simulink model "modificar_acc_compilar"  (R2013b)
settings: Solver=ode45  StartTime=0.0  StopTime=17000  RelTol=1e-3
undefined symbols (not defined in the file): internal_oor, misc_lib, pfb_coeff_gen_calc, xlfda_numerator, xlipgetpartsetting
libraries: xbsIndex_r4 x1539, xps_library x14, dspsigops x8, casper_library_misc x8, casper_library_delays x3, simulink x1
(part 4 of 15)

== system modificar_acc_compilar/acc_cntrl0 ==
  acc_len : Inport
  sync : Inport  Port=2
  rst : Inport  Port=3
  Logical : xbsIndex_r4/Logical  logical_function=OR  inputs=2  en=off  latency=0  precision=Full  arith_type=Unsigned  n_bits=8  bin_pt=2  align_bp=on  dbl_ovrd=off  block_type=logical
      settings: xl_area=[0, 0, 0, 0, 0, 0, 0]
  Register : xbsIndex_r4/Register  init=0  rst=on  en=on  dbl_ovrd=off  block_type=register
      settings: xl_area=[0, 0, 0, 0, 0, 0, 0]
  Relational5 : xbsIndex_r4/Relational  mode=a=b  en=off  latency=0  dbl_ovrd=off  block_type=relational
      settings: xl_area=[0, 0, 0, 0, 0, 0, 0]  block_version=10.1.3
  Shift : xbsIndex_r4/Shift  shift_dir=Left  shift_bits=chan_bits  en=off  latency=0  precision=Full  arith_type="Signed  (2's comp)"  n_bits=8  bin_pt=2  quantization=Truncate  overflow=Wrap  dbl_ovrd=off  block_type=shift
      settings: xl_area=[0, 0, 0, 0, 0, 0, 0]  block_version=10.1.3
  cntr : xbsIndex_r4/Counter  cnt_type=Free Running  cnt_to=Inf  operation=Up  start_count=1  cnt_by_val=1  arith_type=Unsigned  n_bits=32  bin_pt=0  load_pin=off  rst=on  en=off  explicit_period=on  period=1  dbl_ovrd=off  use_behavioral_HDL=on  implementation=Fabric  use_rpm=on  block_type=counter
      settings: xl_area=[0, 0, 0, 0, 0, 0, 0]
  edge_detect : Subsystem  AncestorBlock=casper_library_misc/edge_detect  mask(edge_detect){edge=Rising, polarity=Active High, x_in=[0 0.08 0.08 0.16 0.16 0.24 0.24 0.32 0.32 0.4], y_in=[-1 -1  1  1  1  1  1  1  1  1], x_out=[0.6 0.68 0.68 0.76 0.76 0.84 0.84 0.92 0.92 1], y_out=[-1 -1  1  1 -1 -1 -1 -1 -1 -1]}
      mask prompts: edge "Edge Type"; polarity "Output Polarity"; x_in "Input X Positions"; y_in "Input Y Positions"; x_out "Output X Positions"; y_out "Output Y Positions"
      mask help: Output is active for one-cycle after each edge of the specified type (i.e. rising, falling or both).
      mask init: same as modificar_acc_compilar/edge_detect1
      settings: AttributesFormatString=|
      | rising edges
      | active high
      mask Help: Output is active for one-cycle after each edge of the specified type (i.e. rising, falling, or both).  Latency is zero.
      mask TypeOptions edge: Rising | Falling | Both
      mask TypeOptions polarity: Active High | Active Low
      mask Display:
      | plot(x_in_num,0.5+y_in_num*0.2);
      | plot(x_out_num,0.5+y_out_num*0.2);
  pipeline15 : Subsystem  AncestorBlock=casper_library_delays/pipeline  mask(pipeline){latency=1}
      mask help:
      | An explicitly laid-out delay line to avoid mapping to SRL16s
      | for use in pipelining to help achieve timing closure.
      mask init:
      | pipeline_init(gcb,'latency',latency);
      settings: AttributesFormatString=Latency = %<latency>
      mask Display:
      | port_label('input', 1, 'd');
      | port_label('output', 1, 'q');
      | disp(['Z^-', num2str(latency)]);
  new_acc : Outport
  wires:
  Shift/1 -> pipeline15/1(d)
  rst/1 -> Register/2
  sync/1 -> Register/3, Register/1
  Relational5/1 -> new_acc/1, Logical/2
  acc_len/1 -> Shift/1
  Logical/1 -> cntr/1
  Register/1 -> edge_detect/1(in)
  edge_detect/1(out) -> Logical/1
  pipeline15/1(q) -> Relational5/2
  cntr/1 -> Relational5/1

== system modificar_acc_compilar/acc_len ==
  io_delay : xbsIndex_r4/Delay  rst=off  infoeditControl=Selection of Reset will increase slice count due to use of real FFs and instead of SRLs  en=off  latency=0  dbl_ovrd=off  reg_retiming=on  block_type=delay
  modificar_acc_compilar_acc_len_user_data_out : xbsIndex_r4/Gateway In  gui_display_data_type=Fixed-point  arith_type=Unsigned  n_bits=32  bin_pt=0  preci_type=Single  exp_width=8  frac_width=24  quantization="Round  (unbiased: +/- Inf)"  overflow=Saturate  period=1  dbl_ovrd=off  timing_constraint=None  locs_specified=off  LOCs={}  UseAsADC=off  ADCChannel='1'  inherit_from_input=off  hdl_port=on  block_type=gatewayin
  reint1 : xbsIndex_r4/Reinterpret  force_arith_type=on  arith_type=Unsigned  force_bin_pt=on  bin_pt=0  block_type=reinterpret
  sim_1 : Constant  Value=0
  slice_reg : xbsIndex_r4/Slice  nbits=32  boolean_output=off  mode=Lower Bit Location + Width  bit1=0  base1=MSB of Input  bit0=0  base0=LSB of Input  dbl_ovrd=off  block_type=slice
  in_reg : Outport
  wires:
  modificar_acc_compilar_acc_len_user_data_out/1 -> io_delay/1
  sim_1/1 -> modificar_acc_compilar_acc_len_user_data_out/1
  io_delay/1 -> slice_reg/1
  slice_reg/1 -> reint1/1
  reint1/1 -> in_reg/1

== system modificar_acc_compilar/adc083000x2 ==
  adc0_sync_sim : Inport
  adc0_data_valid_sim : Inport  Port=2
  sim_adc0_data_in : Inport  Port=3
  adc0_sim : Subsystem  AncestorBlock=xps_library/ADCs/adc_sim  mask(adc_sim){nStreams=8, bit_width=8}
      mask prompts: nStreams "Number of Output Streams"; bit_width "Sample Bit Width"
      mask help:
      | This block simulates the behavior of a demuxed ADC, which takes
      | as input a waveform and returns digital samples in parallel at
      | a slower rate.
      |
      | This block is used to simulate the behavior
      mask init:
      | adc_sim_init(gcb, ...
      |     'nStreams', nStreams, ...
      |     'bit_width', bit_width);
  modificar_acc_compilar_adc083000x2_adc0_user_data_valid : xbsIndex_r4/Gateway In  gui_display_data_type=Fixed-point  arith_type=Unsigned  n_bits=1  bin_pt=0  preci_type=Single  exp_width=8  frac_width=24  quantization="Round  (unbiased: +/- Inf)"  overflow=Saturate  period=1  dbl_ovrd=off  timing_constraint=None  locs_specified=off  LOCs={}  UseAsADC=off  ADCChannel='1'  inherit_from_input=off  hdl_port=on  block_type=gatewayin
  modificar_acc_compilar_adc083000x2_adc0_user_outofrange : xbsIndex_r4/Gateway In  gui_display_data_type=Fixed-point  arith_type=Unsigned  n_bits=4  bin_pt=0  preci_type=Single  exp_width=8  frac_width=24  quantization="Round  (unbiased: +/- Inf)"  overflow=Saturate  period=1  dbl_ovrd=off  timing_constraint=None  locs_specified=off  LOCs={}  UseAsADC=off  ADCChannel='1'  inherit_from_input=off  hdl_port=on  block_type=gatewayin
  modificar_acc_compilar_adc083000x2_adc0_user_s{0..7} (8 alike) : xbsIndex_r4/Gateway In  gui_display_data_type=Fixed-point  arith_type=Unsigned  n_bits=8  bin_pt=0  preci_type=Single  exp_width=8  frac_width=24  quantization="Round  (unbiased: +/- Inf)"  overflow=Saturate  period=1  dbl_ovrd=off  timing_constraint=None  locs_specified=off  LOCs={}  UseAsADC=off  ADCChannel='1'  inherit_from_input=off  hdl_port=on  block_type=gatewayin
  modificar_acc_compilar_adc083000x2_adc0_user_s0_conv : xps_library/ADCs/conv  bit_width=8
  modificar_acc_compilar_adc083000x2_adc0_user_s1_conv : xps_library/ADCs/conv  bit_width=8
  modificar_acc_compilar_adc083000x2_adc0_user_s2_conv : xps_library/ADCs/conv  bit_width=8
  modificar_acc_compilar_adc083000x2_adc0_user_s3_conv : xps_library/ADCs/conv  bit_width=8
  modificar_acc_compilar_adc083000x2_adc0_user_s4_conv : xps_library/ADCs/conv  bit_width=8
  modificar_acc_compilar_adc083000x2_adc0_user_s5_conv : xps_library/ADCs/conv  bit_width=8
  modificar_acc_compilar_adc083000x2_adc0_user_s6_conv : xps_library/ADCs/conv  bit_width=8
  modificar_acc_compilar_adc083000x2_adc0_user_s7_conv : xps_library/ADCs/conv  bit_width=8
  modificar_acc_compilar_adc083000x2_adc0_user_sync : xbsIndex_r4/Gateway In  gui_display_data_type=Fixed-point  arith_type=Unsigned  n_bits=4  bin_pt=0  preci_type=Single  exp_width=8  frac_width=24  quantization="Round  (unbiased: +/- Inf)"  overflow=Saturate  period=1  dbl_ovrd=off  timing_constraint=None  locs_specified=off  LOCs={}  UseAsADC=off  ADCChannel='1'  inherit_from_input=off  hdl_port=on  block_type=gatewayin
  adc0_s0 : Outport
  adc0_s1 : Outport  Port=2
  adc0_s2 : Outport  Port=3
  adc0_s3 : Outport  Port=4
  adc0_s4 : Outport  Port=5
  adc0_s5 : Outport  Port=6
  adc0_s6 : Outport  Port=7
  adc0_s7 : Outport  Port=8
  adc0_sync : Outport  Port=9
  adc0_outofrange : Outport  Port=10
  adc0_data_valid : Outport  Port=11
  wires:
  sim_adc0_data_in/1 -> adc0_sim/1(sim_adc_data_in)
  adc0_sim/1(s0) -> modificar_acc_compilar_adc083000x2_adc0_user_s0/1
  modificar_acc_compilar_adc083000x2_adc0_user_s0/1 -> modificar_acc_compilar_adc083000x2_adc0_user_s0_conv/1
  modificar_acc_compilar_adc083000x2_adc0_user_s0_conv/1 -> adc0_s0/1
  adc0_sim/2(s1) -> modificar_acc_compilar_adc083000x2_adc0_user_s1/1
  modificar_acc_compilar_adc083000x2_adc0_user_s1/1 -> modificar_acc_compilar_adc083000x2_adc0_user_s1_conv/1
  modificar_acc_compilar_adc083000x2_adc0_user_s1_conv/1 -> adc0_s1/1
  adc0_sim/3(s2) -> modificar_acc_compilar_adc083000x2_adc0_user_s2/1
  modificar_acc_compilar_adc083000x2_adc0_user_s2/1 -> modificar_acc_compilar_adc083000x2_adc0_user_s2_conv/1
  modificar_acc_compilar_adc083000x2_adc0_user_s2_conv/1 -> adc0_s2/1
  adc0_sim/4(s3) -> modificar_acc_compilar_adc083000x2_adc0_user_s3/1
  modificar_acc_compilar_adc083000x2_adc0_user_s3/1 -> modificar_acc_compilar_adc083000x2_adc0_user_s3_conv/1
  modificar_acc_compilar_adc083000x2_adc0_user_s3_conv/1 -> adc0_s3/1
  adc0_sim/5(s4) -> modificar_acc_compilar_adc083000x2_adc0_user_s4/1
  modificar_acc_compilar_adc083000x2_adc0_user_s4/1 -> modificar_acc_compilar_adc083000x2_adc0_user_s4_conv/1
  modificar_acc_compilar_adc083000x2_adc0_user_s4_conv/1 -> adc0_s4/1
  adc0_sim/6(s5) -> modificar_acc_compilar_adc083000x2_adc0_user_s5/1
  modificar_acc_compilar_adc083000x2_adc0_user_s5/1 -> modificar_acc_compilar_adc083000x2_adc0_user_s5_conv/1
  modificar_acc_compilar_adc083000x2_adc0_user_s5_conv/1 -> adc0_s5/1
  adc0_sim/7(s6) -> modificar_acc_compilar_adc083000x2_adc0_user_s6/1
  modificar_acc_compilar_adc083000x2_adc0_user_s6/1 -> modificar_acc_compilar_adc083000x2_adc0_user_s6_conv/1
  modificar_acc_compilar_adc083000x2_adc0_user_s6_conv/1 -> adc0_s6/1
  adc0_sim/8(s7) -> modificar_acc_compilar_adc083000x2_adc0_user_s7/1
  modificar_acc_compilar_adc083000x2_adc0_user_s7/1 -> modificar_acc_compilar_adc083000x2_adc0_user_s7_conv/1
  modificar_acc_compilar_adc083000x2_adc0_user_s7_conv/1 -> adc0_s7/1
  adc0_sync_sim/1 -> modificar_acc_compilar_adc083000x2_adc0_user_sync/1
  modificar_acc_compilar_adc083000x2_adc0_user_sync/1 -> adc0_sync/1
  adc0_sim/9(of) -> modificar_acc_compilar_adc083000x2_adc0_user_outofrange/1
  modificar_acc_compilar_adc083000x2_adc0_user_outofrange/1 -> adc0_outofrange/1
  adc0_data_valid_sim/1 -> modificar_acc_compilar_adc083000x2_adc0_user_data_valid/1
  modificar_acc_compilar_adc083000x2_adc0_user_data_valid/1 -> adc0_data_valid/1

== system modificar_acc_compilar/adcsnap0 ==
  note: Generate stop
      | when in circular
      | capture mode
  note: Delay start
      | of capture
  note: ctrl:
      | bit0: Put a posedge here
      |         to enable a new capture.
      | bit1: ignore external trigger
      |         and trigger immediately.
      | bit2: ignore external write
      |         enable and capture on
      |         every FPGA clock.
      | bit3: continuously capture
      |         data until we get an
      |         external stop command.
  note: Offset in vector
      | from first element
      | captured, used
      | during circular capture
  note: Number of
      | bytes in
      | buffer and
      | done bit
  note: Number of valid
      | data samples to
      | skip after trigger
      | before starting
      | capture
  note: Value on vin
      | aligned with
      | first sample on
      | din captured
  din : Inport
  we : Inport  Port=2
  trig : Inport  Port=3
  add_del : xbsIndex_r4/Delay  rst=off  infoeditControl=Selection of Reset will increase slice count due to use of real FFs and instead of SRLs  en=off  latency=1  dbl_ovrd=off  reg_retiming=on  block_type=delay
      settings: block_version=11.4
  add_gen : Subsystem  AncestorBlock=casper_library_scopes/snapshot/add_gen  mask{counter_size=10+3+1, increment=8, nsamples=10, burst_size=0, use_dsp48=on}
      mask prompts: counter_size "Address counter size (2^?)"; increment "Address counter increment"; nsamples "Number of samples (2^?)"; burst_size "Burst size (2^?)"; use_dsp48 "dsp48 counter/s"
      mask init:
      | set_param(gcb,'LinkStatus','inactive');
      | if strcmp(use_dsp48,'on'),
      |     set_param([gcb,'/add_gen'],'implementation','DSP48');
      | else
      |     set_param([gcb,'/add_gen'],'implementation','Fabric');
      | end
  basic_ctrl : Subsystem  AncestorBlock=casper_library_scopes/snapshot/basic_ctrl  mask{dram=off, data_width=64}
      mask prompts: data_width "data width"
      mask init:
      | set_param(gcb,'LinkStatus','inactive');
      | set_param([gcb,'/dram_munge'], 'dram', dram);
  bram : Subsystem  Tag=xps:bram  AncestorBlock=xps_library/Shared_BRAM  mask{arith_type=Unsigned, addr_width=10, data_width=64, reg_prim_output=off, reg_core_output=off, optimization=Minimum_Area, data_bin_pt=0, init_vals=[0:2^10-1], sample_rate=1}
      mask prompts: arith_type "Output Data Type"; addr_width "Address width"; data_width "Data Width"; reg_prim_output "Register Primitive Output"; reg_core_output "Register Core Output"; data_bin_pt "Data Binary Point"; init_vals "Initial values (simulation only)"; sample_rate "Sample rate"
      mask init:
      | shared_bram_mask;
      mask TypeOptions arith_type: Unsigned | Signed  (2's comp)
      mask TypeOptions data_width: 8 | 16 | 32 | 64 | 128
      mask TypeOptions optimization: Minimum_Area | Low_Power
  cast : xbsIndex_r4/Convert  gui_display_data_type=Fixed-point  arith_type=Unsigned  n_bits=64  bin_pt=0  float_type=Single  exp_bits=8  fraction_bits=24  quantization=Truncate  overflow=Wrap  en=off  latency=0  dbl_ovrd=off  pipeline=off  block_type=convert
      settings: block_version=11.4
  const0 : Constant  Value=0
  const1 : Constant  Value=10
  ctrl : Subsystem  Tag=xps:sw_reg  AncestorBlock=xps_library/software_register  mask(swreg){io_dir=From Processor, io_delay=0, sample_period=1, names=reg, bitwidths=32, bin_pts=0, arith_types=0, sim_port=on, show_format=on}
      mask prompts: io_dir "I/O direction"; io_delay "I/O delay"; sample_period "Sample period"; names "Bitfield names [msb...lsb]"; bitwidths "Bitfield widths"; bin_pts "Bitfield binary pts"; arith_types "Bitfield types, ufix=0, fix=1, bool=2"; sim_port "Provide sim input/output?"; show_format "Print format string?"
      mask help: A 32-bit software-accessible register. Can be divided into bitfields of varying widths and types using the fields in the block mask.
      mask init:
      | try
      |     swreg_init(gcb)
      | catch ex
      |     disp(sprintf('%s: %s', gcb, ex.message))
      |     errordlg(ex.message)
      | end
      settings: AttributesFormatString=1input:uf32.0 = 32 bits
      mask TypeOptions io_dir: To Processor | From Processor
      mask Callback io_dir:
      | mask_enables = get_param(gcb, 'MaskEnables');
      | mask_names = get_param(gcb, 'MaskNames');
      | if strcmp(get_param(gcb, 'io_dir'), 'To Processor'),
      |     mask_enables{ismember(mask_names, 'sample_period')} = 'off';
      | else
      |     mask_enables{ismember(mask_names, 'sample_period')} = 'on';
      | end
      | set_param(gcb, 'MaskEnables', mask_enables);
  dat_del : xbsIndex_r4/Delay  rst=off  infoeditControl=Selection of Reset will increase slice count due to use of real FFs and instead of SRLs  en=off  latency=1  dbl_ovrd=off  reg_retiming=on  block_type=delay
      settings: block_version=11.4
  delay : Subsystem  AncestorBlock=casper_library_scopes/snapshot/delay  mask{use_dsp48=on, word_size=8}
      mask prompts: use_dsp48 "dsp48 counter/s"; word_size "word byte size?"
      mask init:
      | set_param(gcb,'LinkStatus','inactive');
      | if strcmp(use_dsp48,'on'),
      |     set_param([gcb,'/counter'],'implementation','DSP48');
      | else
      |     set_param([gcb,'/counter'],'implementation','Fabric');
      | end
  g_tr_en_cnt : Terminator
  gbram : Terminator
  gstatus : Terminator
  gval : Terminator
  never : xbsIndex_r4/Constant  const=0  gui_display_data_type=Fixed-point  arith_type=Boolean  n_bits=16  bin_pt=14  preci_type=Single  exp_width=8  frac_width=24  explicit_period=on  period=1  equ=P=C  opselect=C  inp2=PCIN>>17  opr=+  inp1=P  carry=CIN  dbl_ovrd=off  block_type=constant
  ri : xbsIndex_r4/Reinterpret  force_arith_type=on  arith_type=Unsigned  force_bin_pt=on  bin_pt=0  block_type=reinterpret
      settings: infoedit="Changes signal type without altering the binary representation.   You can changed the signal between signed and unsigned, and relocate the binary point.<br><br>Hardware notes: In hardware this block costs nothing.<br><br>Example:  Suppose the input is 6 bits wide, signed, with 2 fractional bits, and the output is forced to unsigned with 0 fractional bits.  Then an input of -2.0 (1110.00 in binary 2's complement) becomes an output of 56 (111000 in binary)."
  status : Subsystem  Tag=xps:sw_reg  AncestorBlock=xps_library/software_register  mask(swreg){io_dir=To Processor, io_delay=0, sample_period=1, names=reg, bitwidths=32, bin_pts=0, arith_types=0, sim_port=on, show_format=on}
      mask prompts: io_dir "I/O direction"; io_delay "I/O delay"; sample_period "Sample period"; names "Bitfield names [msb...lsb]"; bitwidths "Bitfield widths"; bin_pts "Bitfield binary pts"; arith_types "Bitfield types, ufix=0, fix=1, bool=2"; sim_port "Provide sim input/output?"; show_format "Print format string?"
      mask help: A 32-bit software-accessible register. Can be divided into bitfields of varying widths and types using the fields in the block mask.
      mask init:
      | try
      |     swreg_init(gcb)
      | catch ex
      |     disp(sprintf('%s: %s', gcb, ex.message))
      |     errordlg(ex.message)
      | end
      settings: AttributesFormatString=1output:uf32.0 = 32 bits
      mask TypeOptions io_dir: To Processor | From Processor
      mask Callback io_dir:
      | mask_enables = get_param(gcb, 'MaskEnables');
      | mask_names = get_param(gcb, 'MaskNames');
      | if strcmp(get_param(gcb, 'io_dir'), 'To Processor'),
      |     mask_enables{ismember(mask_names, 'sample_period')} = 'off';
      | else
      |     mask_enables{ismember(mask_names, 'sample_period')} = 'on';
      | end
      | set_param(gcb, 'MaskEnables', mask_enables);
  trig_offset : Subsystem  Tag=xps:sw_reg  AncestorBlock=xps_library/software_register  mask(swreg){io_dir=From Processor, io_delay=0, sample_period=1, names=reg, bitwidths=32, bin_pts=0, arith_types=0, sim_port=on, show_format=on}
      mask prompts: io_dir "I/O direction"; io_delay "I/O delay"; sample_period "Sample period"; names "Bitfield names [msb...lsb]"; bitwidths "Bitfield widths"; bin_pts "Bitfield binary pts"; arith_types "Bitfield types, ufix=0, fix=1, bool=2"; sim_port "Provide sim input/output?"; show_format "Print format string?"
      mask help: A 32-bit software-accessible register. Can be divided into bitfields of varying widths and types using the fields in the block mask.
      mask init:
      | try
      |     swreg_init(gcb)
      | catch ex
      |     disp(sprintf('%s: %s', gcb, ex.message))
      |     errordlg(ex.message)
      | end
      settings: AttributesFormatString=1input:uf32.0 = 32 bits
      mask TypeOptions io_dir: To Processor | From Processor
      mask Callback io_dir:
      | mask_enables = get_param(gcb, 'MaskEnables');
      | mask_names = get_param(gcb, 'MaskNames');
      | if strcmp(get_param(gcb, 'io_dir'), 'To Processor'),
      |     mask_enables{ismember(mask_names, 'sample_period')} = 'off';
      | else
      |     mask_enables{ismember(mask_names, 'sample_period')} = 'on';
      | end
      | set_param(gcb, 'MaskEnables', mask_enables);
  vin_const : xbsIndex_r4/Constant  const=0  gui_display_data_type=Fixed-point  arith_type=Boolean  n_bits=16  bin_pt=14  preci_type=Single  exp_width=8  frac_width=24  explicit_period=on  period=1  equ=P=C  opselect=C  inp2=PCIN>>17  opr=+  inp1=P  carry=CIN  dbl_ovrd=off  block_type=constant
  we_del : xbsIndex_r4/Delay  rst=off  infoeditControl=Selection of Reset will increase slice count due to use of real FFs and instead of SRLs  en=off  latency=1  dbl_ovrd=off  reg_retiming=on  block_type=delay
      settings: block_version=11.4
  wires:
  din/1 -> ri/1
  ri/1 -> cast/1
  cast/1 -> basic_ctrl/2(din)
  we/1 -> basic_ctrl/3(we)
  trig/1 -> basic_ctrl/4(trig)
  never/1 -> basic_ctrl/6(stopi)
  const0/1 -> ctrl/1(sim_1)
  ctrl/1(in_reg) -> basic_ctrl/5(ctrl)
  const1/1 -> trig_offset/1(sim_1)
  basic_ctrl/1(vout) -> delay/1(vin)
  basic_ctrl/2(dout) -> delay/2(din)
  basic_ctrl/3(we_o) -> delay/3(we)
  basic_ctrl/4(go) -> delay/4(go)
  basic_ctrl/5(stop) -> delay/5(stopi)
  basic_ctrl/6(init) -> delay/6(init)
  trig_offset/1(in_reg) -> delay/7(delay)
  delay/1(vout) -> add_gen/1(vin)
  delay/2(dout) -> add_gen/2(din)
  delay/3(we_o) -> add_gen/3(we)
  delay/4(del_go) -> add_gen/4(go)
  delay/5(stop) -> add_gen/5(cont)
  delay/6(del_init) -> add_gen/6(init)
  add_gen/5(status) -> status/1(out_reg)
  status/1(sim_out) -> gstatus/1
  vin_const/1 -> basic_ctrl/1(vin)
  add_gen/1(vout) -> gval/1
  add_gen/6(en_cnt) -> g_tr_en_cnt/1
  add_gen/2(add) -> add_del/1
  add_gen/3(dout) -> dat_del/1
  add_gen/4(we_o) -> we_del/1
  add_del/1 -> bram/1(addr)
  dat_del/1 -> bram/2(data_in)
  we_del/1 -> bram/3(we)
  bram/1(data_out) -> gbram/1

== system modificar_acc_compilar/bus_create ==
  in1 : Inport
  in2 : Inport  Port=2
  in3 : Inport  Port=3
  in4 : Inport  Port=4
  in5 : Inport  Port=5
  in6 : Inport  Port=6
  in7 : Inport  Port=7
  in8 : Inport  Port=8
  concatenate : xbsIndex_r4/Concat  num_inputs=8  dbl_ovrd=off  block_type=concat
  reinterpret{1..8} (8 alike) : xbsIndex_r4/Reinterpret  force_arith_type=on  arith_type=Unsigned  force_bin_pt=on  bin_pt=0  block_type=reinterpret
      reinterpret1 settings: infoedit="Changes signal type without altering the binary representation.   You can changed the signal between signed and unsigned, and relocate the binary point.<br><br>Hardware notes: In hardware this block costs nothing.<br><br>Example:  Suppose the input is 6 bits wide, signed, with 2 fractional bits, and the output is forced to unsigned with 0 fractional bits.  Then an input of -2.0 (1110.00 in binary 2's complement) becomes an output of 56 (111000 in binary)."
      reinterpret2 settings: infoedit="Changes signal type without altering the binary representation.   You can changed the signal between signed and unsigned, and relocate the binary point.<br><br>Hardware notes: In hardware this block costs nothing.<br><br>Example:  Suppose the input is 6 bits wide, signed, with 2 fractional bits, and the output is forced to unsigned with 0 fractional bits.  Then an input of -2.0 (1110.00 in binary 2's complement) becomes an output of 56 (111000 in binary)."
  bus_out : Outport
  wires:
  concatenate/1 -> bus_out/1
  in1/1 -> reinterpret1/1
  reinterpret1/1 -> concatenate/1
  in2/1 -> reinterpret2/1
  reinterpret2/1 -> concatenate/2
  in3/1 -> reinterpret3/1
  reinterpret3/1 -> concatenate/3
  in4/1 -> reinterpret4/1
  reinterpret4/1 -> concatenate/4
  in5/1 -> reinterpret5/1
  reinterpret5/1 -> concatenate/5
  in6/1 -> reinterpret6/1
  reinterpret6/1 -> concatenate/6
  in7/1 -> reinterpret7/1
  reinterpret7/1 -> concatenate/7
  in8/1 -> reinterpret8/1
  reinterpret8/1 -> concatenate/8

== system modificar_acc_compilar/cnt_rst ==
  io_delay : xbsIndex_r4/Delay  rst=off  infoeditControl=Selection of Reset will increase slice count due to use of real FFs and instead of SRLs  en=off  latency=0  dbl_ovrd=off  reg_retiming=on  block_type=delay
  modificar_acc_compilar_cnt_rst_user_data_out : xbsIndex_r4/Gateway In  gui_display_data_type=Fixed-point  arith_type=Unsigned  n_bits=32  bin_pt=0  preci_type=Single  exp_width=8  frac_width=24  quantization="Round  (unbiased: +/- Inf)"  overflow=Saturate  period=1  dbl_ovrd=off  timing_constraint=None  locs_specified=off  LOCs={}  UseAsADC=off  ADCChannel='1'  inherit_from_input=off  hdl_port=on  block_type=gatewayin
  reint1 : xbsIndex_r4/Reinterpret  force_arith_type=on  arith_type=Unsigned  force_bin_pt=on  bin_pt=0  block_type=reinterpret
  sim_1 : Constant  Value=0
  slice_reg : xbsIndex_r4/Slice  nbits=32  boolean_output=off  mode=Lower Bit Location + Width  bit1=0  base1=MSB of Input  bit0=0  base0=LSB of Input  dbl_ovrd=off  block_type=slice
  in_reg : Outport
  wires:
  modificar_acc_compilar_cnt_rst_user_data_out/1 -> io_delay/1
  sim_1/1 -> modificar_acc_compilar_cnt_rst_user_data_out/1
  io_delay/1 -> slice_reg/1
  slice_reg/1 -> reint1/1
  reint1/1 -> in_reg/1

== system modificar_acc_compilar/dec_fir ==
  sync_in : Inport
  real1 : Inport  Port=2
  imag1 : Inport  Port=3
  real2 : Inport  Port=4
  imag2 : Inport  Port=5
  real3 : Inport  Port=6
  imag3 : Inport  Port=7
  real4 : Inport  Port=8
  imag4 : Inport  Port=9
  real5 : Inport  Port=10
  imag5 : Inport  Port=11
  real6 : Inport  Port=12
  imag6 : Inport  Port=13
  real7 : Inport  Port=14
  imag7 : Inport  Port=15
  real8 : Inport  Port=16
  imag8 : Inport  Port=17
  convert1 : xbsIndex_r4/Convert  gui_display_data_type=Fixed-point  arith_type="Signed  (2's comp)"  n_bits=8  bin_pt=7  float_type=Single  exp_bits=8  fraction_bits=24  quantization="Round  (unbiased: Even Values)"  overflow=Wrap  en=off  latency=2  dbl_ovrd=off  pipeline=off  block_type=convert
  convert2 : xbsIndex_r4/Convert  gui_display_data_type=Fixed-point  arith_type="Signed  (2's comp)"  n_bits=8  bin_pt=7  float_type=Single  exp_bits=8  fraction_bits=24  quantization="Round  (unbiased: Even Values)"  overflow=Wrap  en=off  latency=2  dbl_ovrd=off  pipeline=off  block_type=convert
  delay : xbsIndex_r4/Delay  rst=off  infoeditControl=Selection of Reset will increase slice count due to use of real FFs and instead of SRLs  en=off  latency=8  dbl_ovrd=off  reg_retiming=off  block_type=delay
  fir_dbl_col1 : Subsystem  AncestorBlock=casper_library_downconverter/fir_dbl_col  mask(fir_dbl_col){n_inputs=8, coeff=[0.0024946   0.0015245  0.00039561 -0.00066997  -0.0014872  -0.0019381   -0.001986  -0.0016732], add_latency=1, mult_latency=2, coeff_bit_width=25, coeff_bin_pt=24, first_stage_hdl=on, adder_imp=DSP48}
      mask prompts: n_inputs "Inputs"; coeff "Coefficients"; add_latency "Add latency"; mult_latency "Mult Latency"; coeff_bit_width "Coefficient bit width"; coeff_bin_pt "Coefficient binary point"; first_stage_hdl "Implement first stage of adder trees on output as behavioural HDL"; adder_imp "Adder implementation"
      mask init:
      | fir_dbl_col_init(gcb, ...
      |     'n_inputs', n_inputs, ...
      |     'coeff', coeff, ...
      |     'mult_latency', mult_latency, ...
      |     'add_latency', add_latency, ...
      |     'coeff_bit_width', coeff_bit_width, ...
      |     'coeff_bin_pt', coeff_bin_pt,  ...
      |     'first_stage_hdl', first_stage_hdl, ...
      |     'adder_imp', adder_imp);
      mask Help: eval('xlWeb(''http://casper.berkeley.edu/wiki/Fir_dbl_col'')')
      mask TypeOptions adder_imp: Behavioral | Fabric | DSP48
  fir_dbl_col2 : Subsystem  AncestorBlock=casper_library_downconverter/fir_dbl_col  mask(fir_dbl_col){n_inputs=8, coeff=[-0.0044931  -0.0034421   -0.001888 -0.00016069   0.0014125    0.002566   0.0031378   0.0030882], add_latency=1, mult_latency=2, coeff_bit_width=25, coeff_bin_pt=24, first_stage_hdl=on, adder_imp=DSP48}
      mask prompts: n_inputs "Inputs"; coeff "Coefficients"; add_latency "Add latency"; mult_latency "Mult Latency"; coeff_bit_width "Coefficient bit width"; coeff_bin_pt "Coefficient binary point"; first_stage_hdl "Implement first stage of adder trees on output as behavioural HDL"; adder_imp "Adder implementation"
      mask init: same as modificar_acc_compilar/dec_fir/fir_dbl_col1
      mask Help: eval('xlWeb(''http://casper.berkeley.edu/wiki/Fir_dbl_col'')')
      mask TypeOptions adder_imp: Behavioral | Fabric | DSP48
  fir_dbl_col3 : Subsystem  AncestorBlock=casper_library_downconverter/fir_dbl_col  mask(fir_dbl_col){n_inputs=8, coeff=[0.0070206   0.0062907   0.0045179   0.0021201 -0.00041502   -0.002623  -0.0041435  -0.0047745], add_latency=1, mult_latency=2, coeff_bit_width=25, coeff_bin_pt=24, first_stage_hdl=on, adder_imp=DSP48}
      mask prompts: n_inputs "Inputs"; coeff "Coefficients"; add_latency "Add latency"; mult_latency "Mult Latency"; coeff_bit_width "Coefficient bit width"; coeff_bin_pt "Coefficient binary point"; first_stage_hdl "Implement first stage of adder trees on output as behavioural HDL"; adder_imp "Adder implementation"
      mask init: same as modificar_acc_compilar/dec_fir/fir_dbl_col1
      mask Help: eval('xlWeb(''http://casper.berkeley.edu/wiki/Fir_dbl_col'')')
      mask TypeOptions adder_imp: Behavioral | Fabric | DSP48
  fir_dbl_col4 : Subsystem  AncestorBlock=casper_library_downconverter/fir_dbl_col  mask(fir_dbl_col){n_inputs=8, coeff=[-0.0099603    -0.01024  -0.0086852  -0.0057578  -0.0021128   0.0015362   0.0045459   0.0064494], add_latency=1, mult_latency=2, coeff_bit_width=25, coeff_bin_pt=24, first_stage_hdl=on, adder_imp=DSP48}
      mask prompts: n_inputs "Inputs"; coeff "Coefficients"; add_latency "Add latency"; mult_latency "Mult Latency"; coeff_bit_width "Coefficient bit width"; coeff_bin_pt "Coefficient binary point"; first_stage_hdl "Implement first stage of adder trees on output as behavioural HDL"; adder_imp "Adder implementation"
      mask init: same as modificar_acc_compilar/dec_fir/fir_dbl_col1
      mask Help: eval('xlWeb(''http://casper.berkeley.edu/wiki/Fir_dbl_col'')')
      mask TypeOptions adder_imp: Behavioral | Fabric | DSP48
  fir_dbl_col5 : Subsystem  AncestorBlock=casper_library_downconverter/fir_dbl_col  mask(fir_dbl_col){n_inputs=8, coeff=[0.013364    0.015916    0.015375    0.012218   0.0073002    0.001672  -0.0036149  -0.0076836], add_latency=1, mult_latency=2, coeff_bit_width=25, coeff_bin_pt=24, first_stage_hdl=on, adder_imp=DSP48}
      mask prompts: n_inputs "Inputs"; coeff "Coefficients"; add_latency "Add latency"; mult_latency "Mult Latency"; coeff_bit_width "Coefficient bit width"; coeff_bin_pt "Coefficient binary point"; first_stage_hdl "Implement first stage of adder trees on output as behavioural HDL"; adder_imp "Adder implementation"
      mask init: same as modificar_acc_compilar/dec_fir/fir_dbl_col1
      mask Help: eval('xlWeb(''http://casper.berkeley.edu/wiki/Fir_dbl_col'')')
      mask TypeOptions adder_imp: Behavioral | Fabric | DSP48
  fir_dbl_col6 : Subsystem  AncestorBlock=casper_library_downconverter/fir_dbl_col  mask(fir_dbl_col){n_inputs=8, coeff=[-0.018626   -0.026826   -0.028907   -0.025732   -0.018733  -0.0096602 -0.00030601   0.0077536], add_latency=1, mult_latency=2, coeff_bit_width=25, coeff_bin_pt=24, first_stage_hdl=on, adder_imp=DSP48}
      mask prompts: n_inputs "Inputs"; coeff "Coefficients"; add_latency "Add latency"; mult_latency "Mult Latency"; coeff_bit_width "Coefficient bit width"; coeff_bin_pt "Coefficient binary point"; first_stage_hdl "Implement first stage of adder trees on output as behavioural HDL"; adder_imp "Adder implementation"
      mask init: same as modificar_acc_compilar/dec_fir/fir_dbl_col1
      mask Help: eval('xlWeb(''http://casper.berkeley.edu/wiki/Fir_dbl_col'')')
      mask TypeOptions adder_imp: Behavioral | Fabric | DSP48
  fir_dbl_col7 : Subsystem  AncestorBlock=casper_library_downconverter/fir_dbl_col  mask(fir_dbl_col){n_inputs=8, coeff=[0.13652     0.12808     0.11213    0.090469    0.065443    0.039684     0.01575  -0.0041933], add_latency=1, mult_latency=2, coeff_bit_width=25, coeff_bin_pt=24, first_stage_hdl=on, adder_imp=DSP48}
      mask prompts: n_inputs "Inputs"; coeff "Coefficients"; add_latency "Add latency"; mult_latency "Mult Latency"; coeff_bit_width "Coefficient bit width"; coeff_bin_pt "Coefficient binary point"; first_stage_hdl "Implement first stage of adder trees on output as behavioural HDL"; adder_imp "Adder implementation"
      mask init: same as modificar_acc_compilar/dec_fir/fir_dbl_col1
      mask Help: eval('xlWeb(''http://casper.berkeley.edu/wiki/Fir_dbl_col'')')
      mask TypeOptions adder_imp: Behavioral | Fabric | DSP48
  imag_sum : Subsystem  AncestorBlock=casper_library_misc/adder_tree  mask(adder_tree){n_inputs=7, latency=1, adder_imp=DSP48, first_stage_hdl=off}
      mask prompts: n_inputs "Number of Inputs"; latency "Add Latency"; adder_imp "Adder implementation"; first_stage_hdl "Use behavioural HDL for first stage of adders"
      mask help:
      | Sums all inputs using a tree of adds and delays.
      |
      | Number of inputs: The number of inputs to the block to be summed
      | Add latency: The number of clock cycles to perform one addition (affects timing)..
      | Adder implementation: choice of fabric or DSP48E core, or behavioral HDL
      | Use behavioural HDL for first stage of adders: Causes the first stage of adders to be absorbed into DSP blocks if multipliers precede them (Virtex 5). Overrides Adder implementation
      mask init:
      | adder_tree_init(gcb, ...
      |     'n_inputs', n_inputs, ...
      |     'latency', latency, ...
      |     'adder_imp', adder_imp, ...
      |     'first_stage_hdl', first_stage_hdl);
      settings: AttributesFormatString=latency 3
      mask Help: eval('xlWeb(''http://casper.berkeley.edu/wiki/Adder_tree'')')
      mask TypeOptions adder_imp: Behavioral | Fabric | DSP48
  real_sum : Subsystem  AncestorBlock=casper_library_misc/adder_tree  mask(adder_tree){n_inputs=7, latency=1, adder_imp=DSP48, first_stage_hdl=off}
      mask prompts: n_inputs "Number of Inputs"; latency "Add Latency"; adder_imp "Adder implementation"; first_stage_hdl "Use behavioural HDL for first stage of adders"
      mask help:
      | Sums all inputs using a tree of adds and delays.
      |
      | Number of inputs: The number of inputs to the block to be summed
      | Add latency: The number of clock cycles to perform one addition (affects timing)..
      | Adder implementation: choice of fabric or DSP48E core, or behavioral HDL
      | Use behavioural HDL for first stage of adders: Causes the first stage of adders to be absorbed into DSP blocks if multipliers precede them (Virtex 5). Overrides Adder implementation
      mask init:
      | adder_tree_init(gcb, ...
      |     'n_inputs', n_inputs, ...
      |     'latency', latency, ...
      |     'adder_imp', adder_imp, ...
      |     'first_stage_hdl', first_stage_hdl);
      settings: AttributesFormatString=latency 3
      mask Help: eval('xlWeb(''http://casper.berkeley.edu/wiki/Adder_tree'')')
      mask TypeOptions adder_imp: Behavioral | Fabric | DSP48
  ri_to_c : casper_library_misc/ri_to_c
  shift1 : xbsIndex_r4/Shift  shift_dir=Left  shift_bits=0  en=off  latency=0  precision=Full  arith_type="Signed  (2's comp)"  n_bits=16  bin_pt=14  quantization=Truncate  overflow=Wrap  dbl_ovrd=off  block_type=shift
  shift2 : xbsIndex_r4/Shift  shift_dir=Left  shift_bits=0  en=off  latency=0  precision=Full  arith_type="Signed  (2's comp)"  n_bits=16  bin_pt=14  quantization=Truncate  overflow=Wrap  dbl_ovrd=off  block_type=shift
  sync_out : Outport
  dout : Outport  Port=2
  wires:
  real1/1 -> fir_dbl_col1/1(real1)
  imag1/1 -> fir_dbl_col1/2(imag1)
  real2/1 -> fir_dbl_col1/3(real2)
  imag2/1 -> fir_dbl_col1/4(imag2)
  real3/1 -> fir_dbl_col1/5(real3)
  imag3/1 -> fir_dbl_col1/6(imag3)
  real4/1 -> fir_dbl_col1/7(real4)
  imag4/1 -> fir_dbl_col1/8(imag4)
  real5/1 -> fir_dbl_col1/9(real5)
  imag5/1 -> fir_dbl_col1/10(imag5)
  real6/1 -> fir_dbl_col1/11(real6)
  imag6/1 -> fir_dbl_col1/12(imag6)
  real7/1 -> fir_dbl_col1/13(real7)
  imag7/1 -> fir_dbl_col1/14(imag7)
  real8/1 -> fir_dbl_col1/15(real8)
  imag8/1 -> fir_dbl_col1/16(imag8)
  fir_dbl_col1/33(real_sum) -> real_sum/2(din1)
  fir_dbl_col1/34(imag_sum) -> imag_sum/2(din1)
  fir_dbl_col1/1(real_out1) -> fir_dbl_col2/1(real1)
  fir_dbl_col1/2(imag_out1) -> fir_dbl_col2/2(imag1)
  fir_dbl_col1/3(real_out2) -> fir_dbl_col2/3(real2)
  fir_dbl_col1/4(imag_out2) -> fir_dbl_col2/4(imag2)
  fir_dbl_col1/5(real_out3) -> fir_dbl_col2/5(real3)
  fir_dbl_col1/6(imag_out3) -> fir_dbl_col2/6(imag3)
  fir_dbl_col1/7(real_out4) -> fir_dbl_col2/7(real4)
  fir_dbl_col1/8(imag_out4) -> fir_dbl_col2/8(imag4)
  fir_dbl_col1/9(real_out5) -> fir_dbl_col2/9(real5)
  fir_dbl_col1/10(imag_out5) -> fir_dbl_col2/10(imag5)
  fir_dbl_col1/11(real_out6) -> fir_dbl_col2/11(real6)
  fir_dbl_col1/12(imag_out6) -> fir_dbl_col2/12(imag6)
  fir_dbl_col1/13(real_out7) -> fir_dbl_col2/13(real7)
  fir_dbl_col1/14(imag_out7) -> fir_dbl_col2/14(imag7)
  fir_dbl_col1/15(real_out8) -> fir_dbl_col2/15(real8)
  fir_dbl_col1/16(imag_out8) -> fir_dbl_col2/16(imag8)
  fir_dbl_col2/33(real_sum) -> real_sum/3(din2)
  fir_dbl_col2/34(imag_sum) -> imag_sum/3(din2)
  fir_dbl_col2/1(real_out1) -> fir_dbl_col3/1(real1)
  fir_dbl_col2/2(imag_out1) -> fir_dbl_col3/2(imag1)
  fir_dbl_col2/3(real_out2) -> fir_dbl_col3/3(real2)
  fir_dbl_col2/4(imag_out2) -> fir_dbl_col3/4(imag2)
  fir_dbl_col2/5(real_out3) -> fir_dbl_col3/5(real3)
  fir_dbl_col2/6(imag_out3) -> fir_dbl_col3/6(imag3)
  fir_dbl_col2/7(real_out4) -> fir_dbl_col3/7(real4)
  fir_dbl_col2/8(imag_out4) -> fir_dbl_col3/8(imag4)
  fir_dbl_col2/9(real_out5) -> fir_dbl_col3/9(real5)
  fir_dbl_col2/10(imag_out5) -> fir_dbl_col3/10(imag5)
  fir_dbl_col2/11(real_out6) -> fir_dbl_col3/11(real6)
  fir_dbl_col2/12(imag_out6) -> fir_dbl_col3/12(imag6)
  fir_dbl_col2/13(real_out7) -> fir_dbl_col3/13(real7)
  fir_dbl_col2/14(imag_out7) -> fir_dbl_col3/14(imag7)
  fir_dbl_col2/15(real_out8) -> fir_dbl_col3/15(real8)
  fir_dbl_col2/16(imag_out8) -> fir_dbl_col3/16(imag8)
  fir_dbl_col3/33(real_sum) -> real_sum/4(din3)
  fir_dbl_col3/34(imag_sum) -> imag_sum/4(din3)
  fir_dbl_col3/1(real_out1) -> fir_dbl_col4/1(real1)
  fir_dbl_col3/2(imag_out1) -> fir_dbl_col4/2(imag1)
  fir_dbl_col3/3(real_out2) -> fir_dbl_col4/3(real2)
  fir_dbl_col3/4(imag_out2) -> fir_dbl_col4/4(imag2)
  fir_dbl_col3/5(real_out3) -> fir_dbl_col4/5(real3)
  fir_dbl_col3/6(imag_out3) -> fir_dbl_col4/6(imag3)
  fir_dbl_col3/7(real_out4) -> fir_dbl_col4/7(real4)
  fir_dbl_col3/8(imag_out4) -> fir_dbl_col4/8(imag4)
  fir_dbl_col3/9(real_out5) -> fir_dbl_col4/9(real5)
  fir_dbl_col3/10(imag_out5) -> fir_dbl_col4/10(imag5)
  fir_dbl_col3/11(real_out6) -> fir_dbl_col4/11(real6)
  fir_dbl_col3/12(imag_out6) -> fir_dbl_col4/12(imag6)
  fir_dbl_col3/13(real_out7) -> fir_dbl_col4/13(real7)
  fir_dbl_col3/14(imag_out7) -> fir_dbl_col4/14(imag7)
  fir_dbl_col3/15(real_out8) -> fir_dbl_col4/15(real8)
  fir_dbl_col3/16(imag_out8) -> fir_dbl_col4/16(imag8)
  fir_dbl_col4/33(real_sum) -> real_sum/5(din4)
  fir_dbl_col4/34(imag_sum) -> imag_sum/5(din4)
  fir_dbl_col4/1(real_out1) -> fir_dbl_col5/1(real1)
  fir_dbl_col4/2(imag_out1) -> fir_dbl_col5/2(imag1)
  fir_dbl_col4/3(real_out2) -> fir_dbl_col5/3(real2)
  fir_dbl_col4/4(imag_out2) -> fir_dbl_col5/4(imag2)
  fir_dbl_col4/5(real_out3) -> fir_dbl_col5/5(real3)
  fir_dbl_col4/6(imag_out3) -> fir_dbl_col5/6(imag3)
  fir_dbl_col4/7(real_out4) -> fir_dbl_col5/7(real4)
  fir_dbl_col4/8(imag_out4) -> fir_dbl_col5/8(imag4)
  fir_dbl_col4/9(real_out5) -> fir_dbl_col5/9(real5)
  fir_dbl_col4/10(imag_out5) -> fir_dbl_col5/10(imag5)
  fir_dbl_col4/11(real_out6) -> fir_dbl_col5/11(real6)
  fir_dbl_col4/12(imag_out6) -> fir_dbl_col5/12(imag6)
  fir_dbl_col4/13(real_out7) -> fir_dbl_col5/13(real7)
  fir_dbl_col4/14(imag_out7) -> fir_dbl_col5/14(imag7)
  fir_dbl_col4/15(real_out8) -> fir_dbl_col5/15(real8)
  fir_dbl_col4/16(imag_out8) -> fir_dbl_col5/16(imag8)
  fir_dbl_col5/33(real_sum) -> real_sum/6(din5)
  fir_dbl_col5/34(imag_sum) -> imag_sum/6(din5)
  fir_dbl_col5/1(real_out1) -> fir_dbl_col6/1(real1)
  fir_dbl_col5/2(imag_out1) -> fir_dbl_col6/2(imag1)
  fir_dbl_col5/3(real_out2) -> fir_dbl_col6/3(real2)
  fir_dbl_col5/4(imag_out2) -> fir_dbl_col6/4(imag2)
  fir_dbl_col5/5(real_out3) -> fir_dbl_col6/5(real3)
  fir_dbl_col5/6(imag_out3) -> fir_dbl_col6/6(imag3)
  fir_dbl_col5/7(real_out4) -> fir_dbl_col6/7(real4)
  fir_dbl_col5/8(imag_out4) -> fir_dbl_col6/8(imag4)
  fir_dbl_col5/9(real_out5) -> fir_dbl_col6/9(real5)
  fir_dbl_col5/10(imag_out5) -> fir_dbl_col6/10(imag5)
  fir_dbl_col5/11(real_out6) -> fir_dbl_col6/11(real6)
  fir_dbl_col5/12(imag_out6) -> fir_dbl_col6/12(imag6)
  fir_dbl_col5/13(real_out7) -> fir_dbl_col6/13(real7)
  fir_dbl_col5/14(imag_out7) -> fir_dbl_col6/14(imag7)
  fir_dbl_col5/15(real_out8) -> fir_dbl_col6/15(real8)
  fir_dbl_col5/16(imag_out8) -> fir_dbl_col6/16(imag8)
  fir_dbl_col6/33(real_sum) -> real_sum/7(din6)
  fir_dbl_col6/34(imag_sum) -> imag_sum/7(din6)
  fir_dbl_col6/1(real_out1) -> fir_dbl_col7/1(real1)
  fir_dbl_col6/2(imag_out1) -> fir_dbl_col7/2(imag1)
  fir_dbl_col6/3(real_out2) -> fir_dbl_col7/3(real2)
  fir_dbl_col6/4(imag_out2) -> fir_dbl_col7/4(imag2)
  fir_dbl_col6/5(real_out3) -> fir_dbl_col7/5(real3)
  fir_dbl_col6/6(imag_out3) -> fir_dbl_col7/6(imag3)
  fir_dbl_col6/7(real_out4) -> fir_dbl_col7/7(real4)
  fir_dbl_col6/8(imag_out4) -> fir_dbl_col7/8(imag4)
  fir_dbl_col6/9(real_out5) -> fir_dbl_col7/9(real5)
  fir_dbl_col6/10(imag_out5) -> fir_dbl_col7/10(imag5)
  fir_dbl_col6/11(real_out6) -> fir_dbl_col7/11(real6)
  fir_dbl_col6/12(imag_out6) -> fir_dbl_col7/12(imag6)
  fir_dbl_col6/13(real_out7) -> fir_dbl_col7/13(real7)
  fir_dbl_col6/14(imag_out7) -> fir_dbl_col7/14(imag7)
  fir_dbl_col6/15(real_out8) -> fir_dbl_col7/15(real8)
  fir_dbl_col6/16(imag_out8) -> fir_dbl_col7/16(imag8)
  fir_dbl_col7/33(real_sum) -> real_sum/8(din7)
  fir_dbl_col7/34(imag_sum) -> imag_sum/8(din7)
  real_sum/2(dout) -> shift1/1
  imag_sum/2(dout) -> shift2/1
  shift1/1 -> convert1/1
  shift2/1 -> convert2/1
  convert1/1 -> ri_to_c/1
  convert2/1 -> ri_to_c/2
  ri_to_c/1 -> dout/1
  sync_in/1 -> delay/1
  delay/1 -> real_sum/1(sync), imag_sum/1(sync)
  real_sum/1(sync_out) -> sync_out/1
  fir_dbl_col2/17(real_back_out1) -> fir_dbl_col1/17(real_back1)
  fir_dbl_col2/18(imag_back_out1) -> fir_dbl_col1/18(imag_back1)
  fir_dbl_col2/19(real_back_out2) -> fir_dbl_col1/19(real_back2)
  fir_dbl_col2/20(imag_back_out2) -> fir_dbl_col1/20(imag_back2)
  fir_dbl_col2/21(real_back_out3) -> fir_dbl_col1/21(real_back3)
  fir_dbl_col2/22(imag_back_out3) -> fir_dbl_col1/22(imag_back3)
  fir_dbl_col2/23(real_back_out4) -> fir_dbl_col1/23(real_back4)
  fir_dbl_col2/24(imag_back_out4) -> fir_dbl_col1/24(imag_back4)
  fir_dbl_col2/25(real_back_out5) -> fir_dbl_col1/25(real_back5)
  fir_dbl_col2/26(imag_back_out5) -> fir_dbl_col1/26(imag_back5)
  fir_dbl_col2/27(real_back_out6) -> fir_dbl_col1/27(real_back6)
  fir_dbl_col2/28(imag_back_out6) -> fir_dbl_col1/28(imag_back6)
  fir_dbl_col2/29(real_back_out7) -> fir_dbl_col1/29(real_back7)
  fir_dbl_col2/30(imag_back_out7) -> fir_dbl_col1/30(imag_back7)
  fir_dbl_col2/31(real_back_out8) -> fir_dbl_col1/31(real_back8)
  fir_dbl_col2/32(imag_back_out8) -> fir_dbl_col1/32(imag_back8)
  fir_dbl_col3/17(real_back_out1) -> fir_dbl_col2/17(real_back1)
  fir_dbl_col3/18(imag_back_out1) -> fir_dbl_col2/18(imag_back1)
  fir_dbl_col3/19(real_back_out2) -> fir_dbl_col2/19(real_back2)
  fir_dbl_col3/20(imag_back_out2) -> fir_dbl_col2/20(imag_back2)
  fir_dbl_col3/21(real_back_out3) -> fir_dbl_col2/21(real_back3)
  fir_dbl_col3/22(imag_back_out3) -> fir_dbl_col2/22(imag_back3)
  fir_dbl_col3/23(real_back_out4) -> fir_dbl_col2/23(real_back4)
  fir_dbl_col3/24(imag_back_out4) -> fir_dbl_col2/24(imag_back4)
  fir_dbl_col3/25(real_back_out5) -> fir_dbl_col2/25(real_back5)
  fir_dbl_col3/26(imag_back_out5) -> fir_dbl_col2/26(imag_back5)
  fir_dbl_col3/27(real_back_out6) -> fir_dbl_col2/27(real_back6)
  fir_dbl_col3/28(imag_back_out6) -> fir_dbl_col2/28(imag_back6)
  fir_dbl_col3/29(real_back_out7) -> fir_dbl_col2/29(real_back7)
  fir_dbl_col3/30(imag_back_out7) -> fir_dbl_col2/30(imag_back7)
  fir_dbl_col3/31(real_back_out8) -> fir_dbl_col2/31(real_back8)
  fir_dbl_col3/32(imag_back_out8) -> fir_dbl_col2/32(imag_back8)
  fir_dbl_col4/17(real_back_out1) -> fir_dbl_col3/17(real_back1)
  fir_dbl_col4/18(imag_back_out1) -> fir_dbl_col3/18(imag_back1)
  fir_dbl_col4/19(real_back_out2) -> fir_dbl_col3/19(real_back2)
  fir_dbl_col4/20(imag_back_out2) -> fir_dbl_col3/20(imag_back2)
  fir_dbl_col4/21(real_back_out3) -> fir_dbl_col3/21(real_back3)
  fir_dbl_col4/22(imag_back_out3) -> fir_dbl_col3/22(imag_back3)
  fir_dbl_col4/23(real_back_out4) -> fir_dbl_col3/23(real_back4)
  fir_dbl_col4/24(imag_back_out4) -> fir_dbl_col3/24(imag_back4)
  fir_dbl_col4/25(real_back_out5) -> fir_dbl_col3/25(real_back5)
  fir_dbl_col4/26(imag_back_out5) -> fir_dbl_col3/26(imag_back5)
  fir_dbl_col4/27(real_back_out6) -> fir_dbl_col3/27(real_back6)
  fir_dbl_col4/28(imag_back_out6) -> fir_dbl_col3/28(imag_back6)
  fir_dbl_col4/29(real_back_out7) -> fir_dbl_col3/29(real_back7)
  fir_dbl_col4/30(imag_back_out7) -> fir_dbl_col3/30(imag_back7)
  fir_dbl_col4/31(real_back_out8) -> fir_dbl_col3/31(real_back8)
  fir_dbl_col4/32(imag_back_out8) -> fir_dbl_col3/32(imag_back8)
  fir_dbl_col5/17(real_back_out1) -> fir_dbl_col4/17(real_back1)
  fir_dbl_col5/18(imag_back_out1) -> fir_dbl_col4/18(imag_back1)
  fir_dbl_col5/19(real_back_out2) -> fir_dbl_col4/19(real_back2)
  fir_dbl_col5/20(imag_back_out2) -> fir_dbl_col4/20(imag_back2)
  fir_dbl_col5/21(real_back_out3) -> fir_dbl_col4/21(real_back3)
  fir_dbl_col5/22(imag_back_out3) -> fir_dbl_col4/22(imag_back3)
  fir_dbl_col5/23(real_back_out4) -> fir_dbl_col4/23(real_back4)
  fir_dbl_col5/24(imag_back_out4) -> fir_dbl_col4/24(imag_back4)
  fir_dbl_col5/25(real_back_out5) -> fir_dbl_col4/25(real_back5)
  fir_dbl_col5/26(imag_back_out5) -> fir_dbl_col4/26(imag_back5)
  fir_dbl_col5/27(real_back_out6) -> fir_dbl_col4/27(real_back6)
  fir_dbl_col5/28(imag_back_out6) -> fir_dbl_col4/28(imag_back6)
  fir_dbl_col5/29(real_back_out7) -> fir_dbl_col4/29(real_back7)
  fir_dbl_col5/30(imag_back_out7) -> fir_dbl_col4/30(imag_back7)
  fir_dbl_col5/31(real_back_out8) -> fir_dbl_col4/31(real_back8)
  fir_dbl_col5/32(imag_back_out8) -> fir_dbl_col4/32(imag_back8)
  fir_dbl_col6/17(real_back_out1) -> fir_dbl_col5/17(real_back1)
  fir_dbl_col6/18(imag_back_out1) -> fir_dbl_col5/18(imag_back1)
  fir_dbl_col6/19(real_back_out2) -> fir_dbl_col5/19(real_back2)
  fir_dbl_col6/20(imag_back_out2) -> fir_dbl_col5/20(imag_back2)
  fir_dbl_col6/21(real_back_out3) -> fir_dbl_col5/21(real_back3)
  fir_dbl_col6/22(imag_back_out3) -> fir_dbl_col5/22(imag_back3)
  fir_dbl_col6/23(real_back_out4) -> fir_dbl_col5/23(real_back4)
  fir_dbl_col6/24(imag_back_out4) -> fir_dbl_col5/24(imag_back4)
  fir_dbl_col6/25(real_back_out5) -> fir_dbl_col5/25(real_back5)
  fir_dbl_col6/26(imag_back_out5) -> fir_dbl_col5/26(imag_back5)
  fir_dbl_col6/27(real_back_out6) -> fir_dbl_col5/27(real_back6)
  fir_dbl_col6/28(imag_back_out6) -> fir_dbl_col5/28(imag_back6)
  fir_dbl_col6/29(real_back_out7) -> fir_dbl_col5/29(real_back7)
  fir_dbl_col6/30(imag_back_out7) -> fir_dbl_col5/30(imag_back7)
  fir_dbl_col6/31(real_back_out8) -> fir_dbl_col5/31(real_back8)
  fir_dbl_col6/32(imag_back_out8) -> fir_dbl_col5/32(imag_back8)
  fir_dbl_col7/17(real_back_out1) -> fir_dbl_col6/17(real_back1)
  fir_dbl_col7/18(imag_back_out1) -> fir_dbl_col6/18(imag_back1)
  fir_dbl_col7/19(real_back_out2) -> fir_dbl_col6/19(real_back2)
  fir_dbl_col7/20(imag_back_out2) -> fir_dbl_col6/20(imag_back2)
  fir_dbl_col7/21(real_back_out3) -> fir_dbl_col6/21(real_back3)
  fir_dbl_col7/22(imag_back_out3) -> fir_dbl_col6/22(imag_back3)
  fir_dbl_col7/23(real_back_out4) -> fir_dbl_col6/23(real_back4)
  fir_dbl_col7/24(imag_back_out4) -> fir_dbl_col6/24(imag_back4)
  fir_dbl_col7/25(real_back_out5) -> fir_dbl_col6/25(real_back5)
  fir_dbl_col7/26(imag_back_out5) -> fir_dbl_col6/26(imag_back5)
  fir_dbl_col7/27(real_back_out6) -> fir_dbl_col6/27(real_back6)
  fir_dbl_col7/28(imag_back_out6) -> fir_dbl_col6/28(imag_back6)
  fir_dbl_col7/29(real_back_out7) -> fir_dbl_col6/29(real_back7)
  fir_dbl_col7/30(imag_back_out7) -> fir_dbl_col6/30(imag_back7)
  fir_dbl_col7/31(real_back_out8) -> fir_dbl_col6/31(real_back8)
  fir_dbl_col7/32(imag_back_out8) -> fir_dbl_col6/32(imag_back8)
  fir_dbl_col7/1(real_out1) -> fir_dbl_col7/17(real_back1)
  fir_dbl_col7/2(imag_out1) -> fir_dbl_col7/18(imag_back1)
  fir_dbl_col7/3(real_out2) -> fir_dbl_col7/19(real_back2)
  fir_dbl_col7/4(imag_out2) -> fir_dbl_col7/20(imag_back2)
  fir_dbl_col7/5(real_out3) -> fir_dbl_col7/21(real_back3)
  fir_dbl_col7/6(imag_out3) -> fir_dbl_col7/22(imag_back3)
  fir_dbl_col7/7(real_out4) -> fir_dbl_col7/23(real_back4)
  fir_dbl_col7/8(imag_out4) -> fir_dbl_col7/24(imag_back4)
  fir_dbl_col7/9(real_out5) -> fir_dbl_col7/25(real_back5)
  fir_dbl_col7/10(imag_out5) -> fir_dbl_col7/26(imag_back5)
  fir_dbl_col7/11(real_out6) -> fir_dbl_col7/27(real_back6)
  fir_dbl_col7/12(imag_out6) -> fir_dbl_col7/28(imag_back6)
  fir_dbl_col7/13(real_out7) -> fir_dbl_col7/29(real_back7)
  fir_dbl_col7/14(imag_out7) -> fir_dbl_col7/30(imag_back7)
  fir_dbl_col7/15(real_out8) -> fir_dbl_col7/31(real_back8)
  fir_dbl_col7/16(imag_out8) -> fir_dbl_col7/32(imag_back8)

== system modificar_acc_compilar/edge_detect1 ==
  in : Inport
  Delay : xbsIndex_r4/Delay  rst=off  infoeditControl=Selection of Reset will increase slice count due to use of real FFs and instead of SRLs  en=off  latency=1  dbl_ovrd=off  reg_retiming=on  block_type=delay
      settings: xl_area=[0, 0, 0, 0, 0, 0, 0]
  Inverter : xbsIndex_r4/Inverter  en=off  latency=0  dbl_ovrd=off  block_type=inv
      settings: xl_area=[0, 0, 0, 0, 0, 0, 0]
  edge_op : xbsIndex_r4/Logical  logical_function=AND  inputs=2  en=off  latency=0  precision=Full  arith_type=Unsigned  n_bits=8  bin_pt=2  align_bp=on  dbl_ovrd=off  block_type=logical
      settings: xl_area=[0, 0, 0, 0, 0, 0, 0]
  out : Outport
  wires:
  Delay/1 -> edge_op/2
  in/1 -> Delay/1, Inverter/1
  edge_op/1 -> out/1
  Inverter/1 -> edge_op/1
